simulink model "Haptic feedbck system"  (R2024b)
settings: Solver=ode4  StartTime=0.0  StopTime=inf  FixedStep=0.001  RelTol=1e-3  EnableMultiTasking=on
undefined symbols (not defined in the file): _, cablePTstudyZF, data, date, DiscIntNeverNeededParam, FETau, HIL, i2tTimeLim, iCmd2Volt, iCmdLim, iCmdSat, iCont, iMeasLim, iMeasServoConv, iPeak, iSign, kDposStudyPC, kDstudyZF, kPposStudyPC, kPstudyZF, kS, magnitude, maxTorque, motEncCnts2Rad, motEncSign, motKt, motNegFfTauStudyPC, motPosFfTauStudyPC, motPulleyRad, pulseGuiPeriod, pulseGuiPulseWidth, qc_get_step_size, signals, sprEncCnts2Rad, sprEncSign, tauDzStudyZF, tauJlim, tauMlim, tauNoMvtStudyZF, test_1_robot_torque_, time, tS, Visualization, xJdotLim, xJlimNeg, xJlimPos, xMdotLim, xMlimNeg, xMlimPos
libraries: quarc_library x26, simulink x13, simulink_extras x2
(part 1 of 3)
settings Model: SimulationMode=external  ExtModeTrigDuration=10000  Creator=Pranav  LastModifiedBy=Pranav
settings SolverCC: AlgebraicLoopSolver=TrustRegion  PositivePriorityOrder=on
settings DataIOCC: ReturnWorkspaceOutputs=off
settings DebuggingCC: UnconnectedInputMsg=warning  UnconnectedOutputMsg=warning  UnconnectedLineMsg=warning  ArithmeticOperatorsInVariantConditions=warning
settings ModelReferenceCC: EnableRefExpFcnMdlSchedulingChecks=on
settings SFSimCC: SimUseLocalCustomCode=off  CustomCodeUndefinedFunction=UseInterfaceOnly
settings RTWCC: Description=QUARC Win64 Target Using Toolchain  SystemTargetFile=quarc_win64.tlc  TemplateMakefile=quarc_default_tmf  RTWUseLocalCustomCode=off  Toolchain=QUARC win64 | nmake (64-bit Windows)  BuildConfiguration=Faster Runs  GPUComputeCapability=3.5
settings CodeAppCC: StateflowObjectComments=on
settings STFCustomTargetCC: TargetLangStandard=C99 (ISO)  ConcurrentExecutionCompliant=on  GRTInterface=on  UseToolchainInfoCompliant=on  SystemTargetFile=quarc_win64.tlc
settings GRTTargetCC: ParMdlRefBuildCompliant=off  CompOptLevelCompliant=off  CombineOutputUpdateFcns=off  MatFileLogging=off  CPPClassGenCompliant=off  GRTInterface=on  ExtMode=on  ExtModeMexFile=quarc_comm
settings ConfigComp: CovMetricSettings=dswe

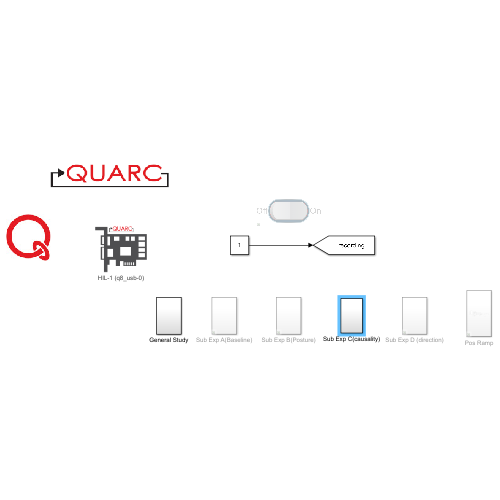
[thumbnail: Simulink's stored preview of the top-level diagram]
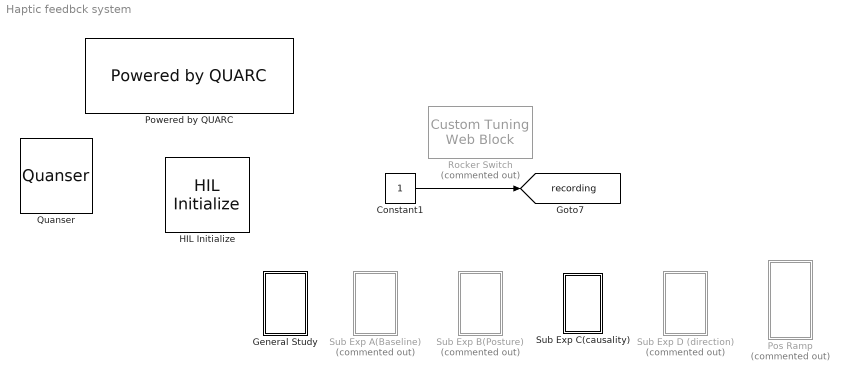
== system Haptic feedbck system ==
  Constant1 : Constant
  General Study : Subsystem
  HIL Initialize : quarc_library/Data Acquisition/Generic/Configuration/HIL Initialize  Priority=-99  object_name=HIL-1  board_type=q8_usb  board_number=0  board_options=update_rate=normal;decimation=1  exclusive=off  active=off  hardware_clocks=[0:2]  clock_modes=[]  initial_clock_frequencies=[]  set_clock_params_at_start=off  set_clock_params_at_switch_in=off  set_clock_frequencies_at_start=off  set_clock_frequencies_at_switch_in=off  analog_input_channels=[0:7]  analog_input_configurations=[]  analog_input_maximums=10  analog_input_minimums=-10  set_analog_input_params_at_start=on  set_analog_input_params_at_switch_in=off  analog_output_channels=[0:7]  analog_output_maximums=10  analog_output_minimums=-10  initial_analog_outputs=[0]  final_analog_outputs=[0]  watchdog_analog_outputs=0  set_analog_output_params_at_start=on  set_analog_output_params_at_switch_in=off  set_analog_outputs_at_start=on  set_analog_outputs_at_switch_in=off  set_analog_outputs_at_terminate=on  set_analog_outputs_at_switch_out=off  set_analog_outputs_on_watchdog=off  digital_input_channels=[]  digital_output_channels=0:7  digital_output_configuration=[]  initial_digital_outputs=[1]  final_digital_outputs=[1]  watchdog_digital_outputs=[0]  set_digital_output_params_at_start=off  set_digital_output_params_at_switch_in=off  set_digital_outputs_at_start=on  set_digital_outputs_at_switch_in=off  set_digital_outputs_at_terminate=on  set_digital_outputs_at_switch_out=off  set_digital_outputs_on_watchdog=off  encoder_channels=[0:7]  quadrature=[4]  encoder_filter_frequency=[]  initial_encoder_counts=[0]  set_encoder_params_at_start=on  set_encoder_params_at_switch_in=off  set_encoder_counts_at_start=off  set_encoder_counts_at_switch_in=off  pwm_channels=[0:7]  pwm_modes=0  pwm_frequency=99.532799999999995e6/4095  pwm_configuration=[0]  pwm_alignment=[0]  pwm_polarity=[1]  pwm_leading_deadband=[0]  pwm_trailing_deadband=[0]  initial_pwm_outputs=[0]  final_pwm_outputs=[0]  watchdog_pwm_outputs=[0]  set_pwm_params_at_start=on  set_pwm_params_at_switch_in=off  set_pwm_outputs_at_start=on  set_pwm_outputs_at_switch_in=off  set_pwm_outputs_at_terminate=on  set_pwm_outputs_at_switch_out=off  set_pwm_outputs_on_watchdog=off  other_output_channels=[]  initial_other_outputs=[]  final_other_outputs=[]  watchdog_other_outputs=[]  set_other_outputs_at_start=off  set_other_outputs_at_switch_in=off  set_other_outputs_at_terminate=off  set_other_outputs_at_switch_out=off  set_other_outputs_on_watchdog=off
  Pos Ramp : Subsystem  Commented=on
  Powered by QUARC : quarc_library/Logos/Powered by QUARC
  Quanser : quarc_library/Logos/Quanser
  Rocker Switch : CustomTuningWebBlock  Commented=on  LabelPosition=Hide  ShowInitialText=on  Configuration="{\"components\":[{\"name\":\"CustomSwitchStateComponent\",\"settings\":{\"position\":[0,0,1,1],\"states\":[{\"HitRegion\":{\"position\":[0,0,0.5,1]},\"Image\":{\"position\":[0.13,0,1,0.75],\"size\":[1,0.75],\"src\":\"data:image\\/svg+xml;base64,PHN2ZyB4bWxucz0iaHR0cDovL3d3dy53My5vcmcvMjAwMC9zdmciIHhtbG5zOnhsaW5rPSJodHRwOi8vd3d3LnczLm9yZy8xOTk5L3hsaW5rIiB2aWV3Qm94PSIwIDAgNzUgMjQuOCI+PGRlZnM+PHN0eWxlPi5jbHMtMXtmaWxsOnVybCgjcmFkaWFsLWdyYWRpZW50KTt9LmNscy0ye2ZpbGw6dXJsKCNyYWRpYWwtZ3JhZGllbnQtMik7fS5jbHMtM3tzdHJva2U6I2IyMDAwMDtzdHJva2Utd2lkdGg6MC4yNXB4O2ZpbGw6dXJsKCNsaW5lYXItZ3JhZGllbnQpO30uY2xzLTR7ZmlsbDp1cmwoI2xpbmVhci1ncmFkaWVudC0yKTt9LmNs ...(+3576 chars)\",\"srcOrientation\":\"Right\"},\"Label\":{\"color\":[0.5019607843137255,0.5019607843137255,0.5019607843137255],\"icon\":{\"size\":[0,0],\"src\":[],\"srcOrientation\":\"Right\"},\"iconPlacement\":\"left\",\"opacity\":1,\"position\":[0.5,0.08],\"show\":true,\"text\":{\"content\":\"Off\",\"font\":\"Helvetica\"}},\"Value\":0},{\"HitRegion\":{\"position\":[0,0.5,0.5,1]},\"Image\":{\"position\":[0.13,0,1,0.75],\"size\":[1,0.75],\"src\":\"data:image\\/svg+xml;base64,PHN2ZyB4bWxucz0iaHR0cDovL3d3dy53My5vcmcvMjAwMC9zdmciIHhtbG5zOnhsaW5rPSJodHRwOi8vd3d3LnczLm9yZy8xOTk5L3hsaW5rIiB2aWV3Qm94PSIwIDAgNzUgMjQuOCI+PGRlZnM+PHN0eWxlPi5jbHMtMXtmaWxsOnVybCgjcmFkaWFsLWdyYWRpZW50KTt9LmNscy0ye2ZpbGw6dXJsKCNyYWRpYWwtZ3JhZGllbnQtMik7fS5jbHMtM3tzdHJva2U6I2IyMDAwMDtzdHJva2Utd2lkdGg6MC4yNXB4O2ZpbGw6dXJsKCNsaW5lYXItZ3JhZGllbnQpO30uY2xzLTR7ZmlsbDp1cmwoI2xpbmVhci1ncmFkaWVudC0yKTt9LmNs ...(+3520 chars)\",\"srcOrientation\":\"Right\"},\"Label\":{\"color\":[0.5019607843137255,0.5019607843137255,0.5019607843137255],\"icon\":{\"size\":[0,0],\"src\":[],\"srcOrientation\":\"Right\"},\"iconPlacement\":\"left\",\"opacity\":1,\"position\":[0.5,0.92],\"show\":true,\"text\":{\"content\":\"On\",\"font\":\"Helvetica\"}},\"Value\":1}]}},{\"name\":\"BackgroundImageComponent\",\"settings\":{\"image\":{\"size\":[155,70],\"src\":\"default\",\"srcOrientation\":\"Right\"},\"position\":[0,0,1,1],\"scaleMode\":\"0\"}},{\"name\":\"ForegroundImageComponent\",\"settings\":{\"image\":{\"size\":[0,0],\"src\":\"default\",\"srcOrientation\":[]},\"isForeground\":1,\"position\":[0,0,1,1],\"scaleMode\":\"0\"}}],\"settings\":{\"BindingType\":\"param\",\"backgroundColor\":[0,0,255,\"1\"],\"backgroundOffset\":0.14,\"fixedAspectRatio\":\"on\",\"foregroundColor\":[234,234,234],\"showBackgroundColor\":false,\"variant\":\"rocker\",\"version\":\"R2024b\"},\"type\":\"Switch\"}"
  Sub Exp A(Baseline) : Subsystem  Commented=on
  Sub Exp B(Posture) : Subsystem  Commented=on
  Sub Exp C(causality) : Subsystem
  Sub Exp D (direction) : Subsystem  Commented=on
  tag scope: recording=global
  wires:
  Constant1/1 -> [recording]

== system Haptic feedbck system/General Study ==
  Calculations : Subsystem
  Enable : Subsystem
  Hardware Enable : Subsystem
  Measurements : Subsystem
  Simulation Stops : Subsystem

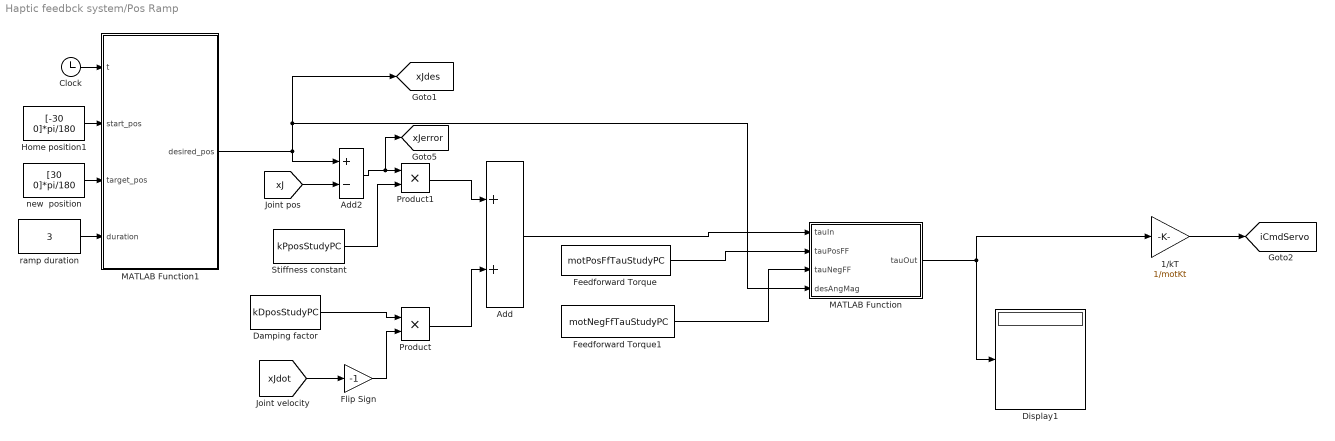
== system Haptic feedbck system/Pos Ramp ==
  1/kT : Gain  Gain=1/motKt
  Add : Sum
  Add2 : Sum  Inputs=+-
  Clock : Clock
  Damping factor : Constant  Value=kDposStudyPC
  Display1 : Display
  Feedforward Torque : Constant  Value=motPosFfTauStudyPC
  Feedforward Torque1 : Constant  Value=motNegFfTauStudyPC
  Flip Sign : Gain  Gain=-1
  Home position1 : Constant  Value=[-30 0]*pi/180
  MATLAB Function : MATLAB Function  TreatAsAtomicUnit=on
  MATLAB Function1 : MATLAB Function  TreatAsAtomicUnit=on
  Product : Product  RndMeth=Zero
  Product1 : Product  RndMeth=Zero
  Stiffness constant : Constant  Value=kPposStudyPC
  new  position : Constant  Value=[30 0]*pi/180
  ramp duration : Constant  Value=3
  tag scope: iCmdServo=global, xJdes=global, xJerror=global
  wires:
  Add2/1 -> [xJerror], Product1/1
  Damping factor/1 -> Product/1
  1/kT/1 -> [iCmdServo]
  Stiffness constant/1 -> Product1/2
  MATLAB Function/1(tauOut) -> Display1/1, 1/kT/1
  Flip Sign/1 -> Product/2
  [xJ] -> Add2/2
  [xJdot] -> Flip Sign/1
  Feedforward Torque1/1 -> MATLAB Function/3(tauNegFF)
  Feedforward Torque/1 -> MATLAB Function/2(tauPosFF)
  Add/1 -> MATLAB Function/1(tauIn)
  Product1/1 -> Add/1
  Product/1 -> Add/2
  MATLAB Function1/1(desired_pos) -> [xJdes], MATLAB Function/4(desAngMag), Add2/1
  new  position/1 -> MATLAB Function1/3(target_pos)
  Clock/1 -> MATLAB Function1/1(t)
  ramp duration/1 -> MATLAB Function1/4(duration)
  Home position1/1 -> MATLAB Function1/2(start_pos)

== system Haptic feedbck system/Sub Exp A(Baseline) ==
  "Active User Control " : Subsystem
  Active User GUI : Subsystem
  Active UserData Recording : Subsystem

== system Haptic feedbck system/Sub Exp B(Posture) ==
  "Active User Control " : Subsystem
  Active User GUI : Subsystem
  Active UserData Recording : Subsystem

== system Haptic feedbck system/Sub Exp C(causality) ==
  Passive User Control : Subsystem
  Passive User GUI : Subsystem
  Passive UserData Recording : Subsystem

== system Haptic feedbck system/Sub Exp D (direction) ==
  "Active User Control " : Subsystem
  Active User GUI : Subsystem
  Active UserData Recording : Subsystem

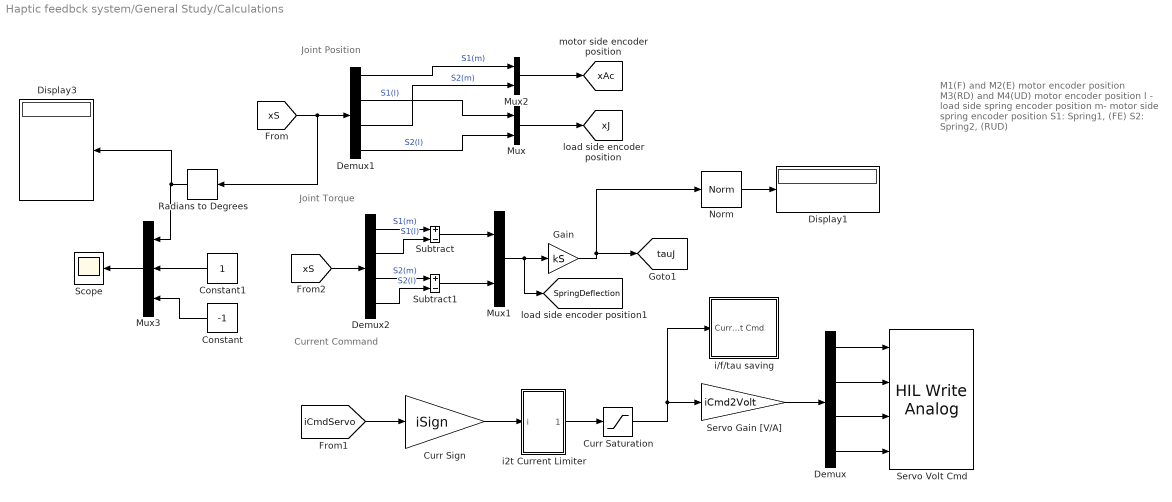
== system Haptic feedbck system/General Study/Calculations ==
  note: M1(F) and M2(E) motor encoder position
      | M3(RD) and M4(UD) motor encoder position
      | l - load side spring encoder position
      | m- motor side spring encoder position
      | S1: Spring1, (FE)
      | S2: Spring2, (RUD)
  note: Joint Position
  note: Joint Torque
  note: Current Command
  Constant : Constant  Value=-1
  Constant1 : Constant
  Curr Saturation : Saturate  UpperLimit=iCmdSat  LowerLimit=-iCmdSat
  Curr Sign : Gain  Gain=iSign
  Demux : Demux
  Demux1 : Demux
  Demux2 : Demux
  Display1 : Display
  Display3 : Display
  Gain : Gain  Gain=kS
  Mux : Mux  Inputs=2
  Mux1 : Mux  Inputs=2
  Mux2 : Mux  Inputs=2
  Mux3 : Mux  Inputs=3
  Norm : quarc_library/Math Operations/Vectors/Norm
      settings: SourceProductName=QUARC Targets
  Radians to Degrees : simulink_extras/Transformations/Radians to Degrees
  Scope : Scope
  Servo Gain [V/A] : Gain  Gain=iCmd2Volt
  Servo Volt Cmd : quarc_library/Data Acquisition/Generic/Immediate I//O/HIL Write Analog  object_name=HIL-1  channels=0:3  sample_time=-1  active=off  vector_input=off
  Subtract : Sum  Inputs=+-
  Subtract1 : Sum  Inputs=+-
  i/f/tau saving : Subsystem
  i2t Current Limiter : Subsystem
  tag scope: SpringDeflection=global, tauJ=global, xAc=global, xJ=global
  wires:
  [xS] -> Radians to Degrees/1, Demux1/1
  Demux1/2 -> Mux/1  "S1(l)"
  Demux1/1 -> Mux2/1  "S1(m)"
  Demux1/4 -> Mux/2  "S2(l)"
  [xS] -> Demux2/1
  Demux2/1 -> Subtract/1  "S1(m)"
  Demux2/2 -> Subtract/2  "S1(l)"
  Demux2/3 -> Subtract1/1  "S2(m)"
  Demux2/4 -> Subtract1/2  "S2(l)"
  Mux1/1 -> [SpringDeflection], Gain/1
  Gain/1 -> Norm/1, [tauJ]
  Demux/1 -> Servo Volt Cmd/1
  Servo Gain [V/A]/1 -> Demux/1
  Curr Saturation/1 -> Servo Gain [V/A]/1, i/f/tau saving/1(Current Cmd)
  Curr Sign/1 -> i2t Current Limiter/1(i)
  Demux/2 -> Servo Volt Cmd/2
  i2t Current Limiter/1(i_lim) -> Curr Saturation/1
  Demux/3 -> Servo Volt Cmd/3
  Demux/4 -> Servo Volt Cmd/4
  Mux/1 -> [xJ]
  Constant1/1 -> Mux3/2
  Mux3/1 -> Scope/1
  Norm/1 -> Display1/1
  Radians to Degrees/1 -> Display3/1, Mux3/1
  Demux1/3 -> Mux2/2  "S2(m)"
  Mux2/1 -> [xAc]
  Subtract/1 -> Mux1/1
  Subtract1/1 -> Mux1/2
  Constant/1 -> Mux3/3
  [iCmdServo] -> Curr Sign/1

== system Haptic feedbck system/General Study/Enable ==
  note: Enable (1 = On, 0 = Off)
  M1 Enable : Constant
  M2 Enable : Constant
  M3 Enable : Constant
  M4 Enable : Constant
  Master  Enable : Constant
  tag scope: M1Enable=global, M2Enable=global, M3Enable=global, M4Enable=global, masterEnable=global
  wires:
  M1 Enable/1 -> [M1Enable]
  Master  Enable/1 -> [masterEnable]
  M2 Enable/1 -> [M2Enable]
  M3 Enable/1 -> [M3Enable]
  M4 Enable/1 -> [M4Enable]

== system Haptic feedbck system/General Study/Hardware Enable ==
  note: Enable/Inhibit Hardware on Servo Amp
      | 0 = Off (GND)
      | 1 = On (+5v)
  note: Hardware Enable
  Gain{1..4} (4 alike) : Gain  Gain=5
  HIL Write Analog : quarc_library/Data Acquisition/Generic/Immediate I//O/HIL Write Analog  object_name=HIL-1  channels=4:7  sample_time=-1  active=off  vector_input=off
  Product{1..4} (4 alike) : Product  RndMeth=Zero
  Saturation{1..4} (4 alike) : Saturate  UpperLimit=5  LowerLimit=0
  wires:
  [M1Enable] -> Product1/1
  Product1/1 -> Gain1/1
  Product2/1 -> Gain2/1
  Saturation1/1 -> HIL Write Analog/1
  Saturation2/1 -> HIL Write Analog/2
  Gain1/1 -> Saturation1/1
  Gain2/1 -> Saturation2/1
  [M2Enable] -> Product2/1
  Product3/1 -> Gain3/1
  Saturation3/1 -> HIL Write Analog/3
  Gain3/1 -> Saturation3/1
  [M3Enable] -> Product3/1
  Product4/1 -> Gain4/1
  Saturation4/1 -> HIL Write Analog/4
  Gain4/1 -> Saturation4/1
  [M4Enable] -> Product4/1
  [masterEnable] -> Product4/2, Product3/2, Product2/2, Product1/2

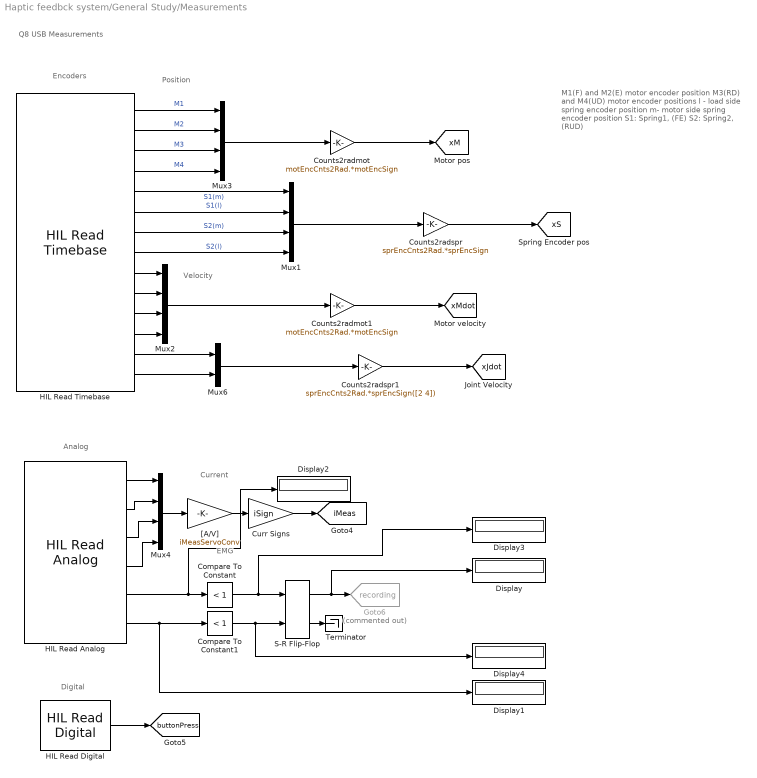
== system Haptic feedbck system/General Study/Measurements ==
  note: M1(F) and M2(E) motor encoder position
      | M3(RD) and M4(UD) motor encoder positions
      | l - load side spring encoder position
      | m- motor side spring encoder position
      | S1: Spring1, (FE)
      | S2: Spring2, (RUD)
  note: Current
  note: Q8 USB Measurements
  note: Encoders
  note: Digital
  note: EMG
  note: Analog
  note: Position
  note: Velocity
  Compare To Constant : simulink/Logic and Bit Operations/Compare To Constant  relop=<  const=1  OutDataTypeStr=boolean
  Compare To Constant1 : simulink/Logic and Bit Operations/Compare To Constant  relop=<  const=1  OutDataTypeStr=boolean
  Counts2radmot : Gain  Gain=motEncCnts2Rad.*motEncSign
  Counts2radmot1 : Gain  Gain=motEncCnts2Rad.*motEncSign
  Counts2radspr : Gain  Gain=sprEncCnts2Rad.*sprEncSign
  Counts2radspr1 : Gain  Gain=sprEncCnts2Rad.*sprEncSign([2 4])
  Curr Signs : Gain  Gain=iSign
  Display{,1..4} (5 alike) : Display
  Goto6 : Goto  Commented=on  GotoTag=recording  TagVisibility=global
  HIL Read Timebase : quarc_library/Data Acquisition/Generic/Timebases/HIL Read Timebase  object_name=HIL-1  clock=0  analog_channels=[]  encoder_channels=[0:7]  digital_channels=[]  other_channels=[14000:14003 14005 14007]  active=on  vector_output=off  data_type_mode=Inherit via back propagation  encoder_data_type=double  digital_data_type=boolean  overflow_mode=Error on overflow  samples_in_buffer=max(ceil(1/qc_get_step_size), 1)
  HIL Read Analog : quarc_library/Data Acquisition/Generic/Immediate I//O/HIL Read Analog  object_name=HIL-1  channels=[0:5]  sample_time=qc_get_step_size  active=on  vector_output=off
  HIL Read Digital : quarc_library/Data Acquisition/Generic/Immediate I//O/HIL Read Digital  object_name=HIL-1  channels=7  sample_time=qc_get_step_size  active=on  vector_output=off  data_type_mode=Inherit via back propagation  data_type=boolean
      settings: AttributesFormatString=(%<object_name>)  SourceProductName=QUARC Targets
  Mux{1..4} (4 alike) : Mux
  Mux6 : Mux  Inputs=2
  S-R Flip-Flop : simulink_extras/Flip Flops/S-R Flip-Flop  initial_condition=0
  Terminator : Terminator
  "[A/V]" : Gain  Gain=iMeasServoConv
  tag scope: buttonPress=global, iMeas=global, xJdot=global, xM=global, xMdot=global, xS=global
  wires:
  Mux3/1 -> Counts2radmot/1
  Counts2radspr/1 -> [xS]
  Counts2radmot/1 -> [xM]
  Mux4/1 -> "[A/V]"/1
  Curr Signs/1 -> [iMeas]
  "[A/V]"/1 -> Curr Signs/1
  HIL Read Analog/1 -> Mux4/1
  HIL Read Analog/2 -> Mux4/2
  HIL Read Analog/3 -> Mux4/3
  HIL Read Analog/4 -> Mux4/4
  Counts2radmot1/1 -> [xMdot]
  Mux2/1 -> Counts2radmot1/1
  HIL Read Digital/1 -> [buttonPress]
  HIL Read Timebase/1 -> Mux3/1  "M1"
  HIL Read Timebase/2 -> Mux3/2  "M2"
  HIL Read Timebase/3 -> Mux3/3  "M3"
  HIL Read Timebase/4 -> Mux3/4  "M4"
  HIL Read Timebase/5 -> Mux1/1  "S1(m)"
  HIL Read Timebase/6 -> Mux1/2  "S1(l)"
  HIL Read Timebase/7 -> Mux1/3  "S2(m)"
  HIL Read Timebase/8 -> Mux1/4  "S2(l)"
  Mux1/1 -> Counts2radspr/1
  HIL Read Timebase/9 -> Mux2/1
  HIL Read Timebase/10 -> Mux2/2
  HIL Read Timebase/11 -> Mux2/3
  HIL Read Timebase/12 -> Mux2/4
  HIL Read Timebase/13 -> Mux6/1
  HIL Read Timebase/14 -> Mux6/2
  Mux6/1 -> Counts2radspr1/1
  Counts2radspr1/1 -> [xJdot]
  Compare To Constant1/1 -> Display4/1, S-R Flip-Flop/2
  HIL Read Analog/5 -> Display2/1, Compare To Constant/1
  S-R Flip-Flop/1 -> Display/1, Goto6/1
  Compare To Constant/1 -> Display3/1, S-R Flip-Flop/1
  S-R Flip-Flop/2 -> Terminator/1
  HIL Read Analog/6 -> Display1/1, Compare To Constant1/1

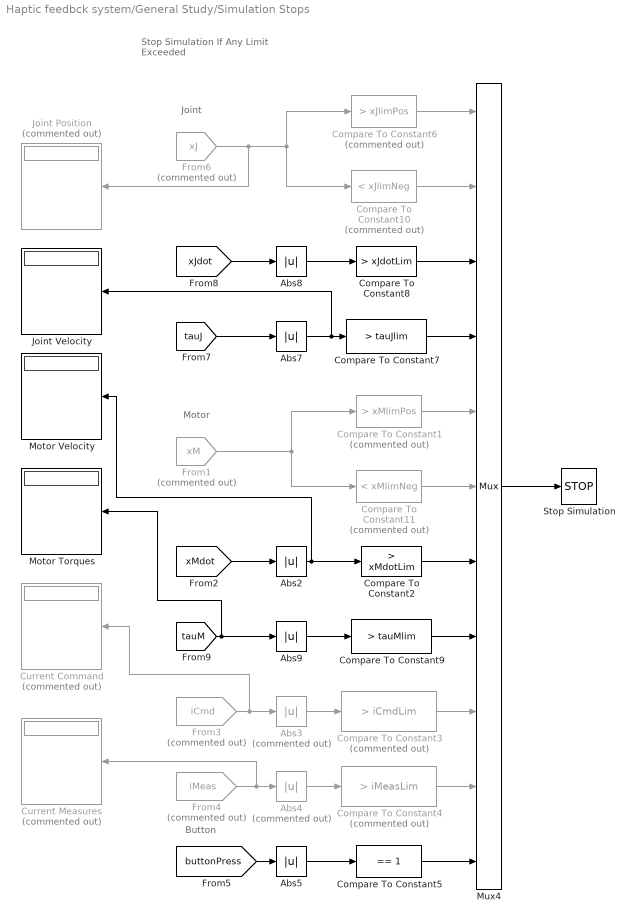
== system Haptic feedbck system/General Study/Simulation Stops ==
  note: Button
  note: Stop Simulation If Any
      | Limit Exceeded
  note: Motor
  note: Joint
  Abs{2,5,7..9} (5 alike) : Abs  SaturateOnIntegerOverflow=off
  Abs3 : Abs  Commented=on  SaturateOnIntegerOverflow=off
  Abs4 : Abs  Commented=on  SaturateOnIntegerOverflow=off
  Compare To Constant1 : simulink/Logic and Bit Operations/Compare To Constant  Commented=on  relop=>  const=xMlimPos  OutDataTypeStr=boolean
  Compare To Constant10 : simulink/Logic and Bit Operations/Compare To Constant  Commented=on  relop=<  const=xJlimNeg  OutDataTypeStr=boolean
  Compare To Constant11 : simulink/Logic and Bit Operations/Compare To Constant  Commented=on  relop=<  const=xMlimNeg  OutDataTypeStr=boolean
  Compare To Constant2 : simulink/Logic and Bit Operations/Compare To Constant  relop=>  const=xMdotLim  OutDataTypeStr=boolean
  Compare To Constant3 : simulink/Logic and Bit Operations/Compare To Constant  Commented=on  relop=>  const=iCmdLim  OutDataTypeStr=boolean
  Compare To Constant4 : simulink/Logic and Bit Operations/Compare To Constant  Commented=on  relop=>  const=iMeasLim  OutDataTypeStr=boolean
  Compare To Constant5 : simulink/Logic and Bit Operations/Compare To Constant  relop===  const=1  OutDataTypeStr=boolean
  Compare To Constant6 : simulink/Logic and Bit Operations/Compare To Constant  Commented=on  relop=>  const=xJlimPos  OutDataTypeStr=boolean
  Compare To Constant7 : simulink/Logic and Bit Operations/Compare To Constant  relop=>  const=tauJlim  OutDataTypeStr=boolean
  Compare To Constant8 : simulink/Logic and Bit Operations/Compare To Constant  relop=>  const=xJdotLim  OutDataTypeStr=boolean
  Compare To Constant9 : simulink/Logic and Bit Operations/Compare To Constant  relop=>  const=tauMlim  OutDataTypeStr=boolean
  Current Command : Display  Commented=on
  Current Measures : Display  Commented=on
  From1 : From  Commented=on  GotoTag=xM  TagVisibility=global
  From3 : From  Commented=on  GotoTag=iCmd  TagVisibility=global
  From4 : From  Commented=on  GotoTag=iMeas  TagVisibility=global
  From6 : From  Commented=on  GotoTag=xJ  TagVisibility=global
  Joint Position : Display  Commented=on
  Joint Velocity : Display
  Motor Torques : Display
  Motor Velocity : Display
  Mux4 : Mux  Inputs=11
  Stop Simulation : Stop
  wires:
  Abs5/1 -> Compare To Constant5/1
  [buttonPress] -> Abs5/1
  Abs3/1 -> Compare To Constant3/1
  From4/1 -> Current Measures/1, Abs4/1
  Abs4/1 -> Compare To Constant4/1
  From1/1 -> Compare To Constant11/1, Compare To Constant1/1
  [tauJ] -> Abs7/1
  Abs7/1 -> Joint Velocity/1, Compare To Constant7/1
  Abs8/1 -> Compare To Constant8/1
  [xJdot] -> Abs8/1
  [tauM] -> Abs9/1, Motor Torques/1
  Abs9/1 -> Compare To Constant9/1
  Abs2/1 -> Compare To Constant2/1, Motor Velocity/1
  [xMdot] -> Abs2/1
  From6/1 -> Joint Position/1, Compare To Constant6/1, Compare To Constant10/1
  Compare To Constant6/1 -> Mux4/1
  Compare To Constant10/1 -> Mux4/2
  Compare To Constant8/1 -> Mux4/3
  Compare To Constant7/1 -> Mux4/4
  Compare To Constant1/1 -> Mux4/5
  Compare To Constant11/1 -> Mux4/6
  Compare To Constant2/1 -> Mux4/7
  Compare To Constant9/1 -> Mux4/8
  Compare To Constant3/1 -> Mux4/9
  Compare To Constant4/1 -> Mux4/10
  Compare To Constant5/1 -> Mux4/11
  Mux4/1 -> Stop Simulation/1
  From3/1 -> Current Command/1, Abs3/1

== system Haptic feedbck system/Sub Exp A(Baseline)/Active User Control  ==
  1/kT : Gain  Gain=1/motKt
  Add : Sum
  Add2 : Sum  Inputs=+-
  Damping factor : Constant  Value=kDposStudyPC
  Display1 : Display
  Feedforward Torque : Constant  Value=motPosFfTauStudyPC
  Feedforward Torque1 : Constant  Value=motNegFfTauStudyPC
  Flip Sign : Gain  Gain=-1
  Home position1 : Constant  Value=[0 0]
  MATLAB Function : MATLAB Function  TreatAsAtomicUnit=on
  Product : Product  RndMeth=Zero
  Product1 : Product  RndMeth=Zero
  Stiffness constant : Constant  Value=kPposStudyPC
  tag scope: iCmdServo=global, xJdes=global, xJerror=global
  wires:
  Add2/1 -> [xJerror], Product1/1
  Damping factor/1 -> Product/1
  1/kT/1 -> [iCmdServo]
  Stiffness constant/1 -> Product1/2
  MATLAB Function/1(tauOut) -> Display1/1, 1/kT/1
  Flip Sign/1 -> Product/2
  [xJ] -> Add2/2
  [xJdot] -> Flip Sign/1
  Feedforward Torque1/1 -> MATLAB Function/3(tauNegFF)
  Feedforward Torque/1 -> MATLAB Function/2(tauPosFF)
  Add/1 -> MATLAB Function/1(tauIn)
  Product1/1 -> Add/1
  Product/1 -> Add/2
  Home position1/1 -> [xJdes], MATLAB Function/4(desAngMag), Add2/1

== system Haptic feedbck system/Sub Exp A(Baseline)/Active User GUI ==
  GUI Triggered Subsytem : Subsystem  TreatAsAtomicUnit=on
  Pulse Generator : DiscretePulseGenerator  PulseType=Time based  Period=pulseGuiPeriod  PulseWidth=pulseGuiPulseWidth
  target angles : Constant  Value=[0 180]*pi/180
  tag scope: FEtau2=global, RUtau2=global, TrialStart2=global, successfulTrial2=global, theta2=global
  wires:
  Pulse Generator/1 -> GUI Triggered Subsytem/Trigger
  target angles/1 -> GUI Triggered Subsytem/2(thetaSel)
  [tauJ] -> GUI Triggered Subsytem/1(tauJ)
  GUI Triggered Subsytem/1(Outport) -> [theta2]
  GUI Triggered Subsytem/2(Outport1) -> [FEtau2]
  GUI Triggered Subsytem/3(Outport2) -> [TrialStart2]
  GUI Triggered Subsytem/4(Outport3) -> [RUtau2]
  GUI Triggered Subsytem/5(Outport5) -> [successfulTrial2]

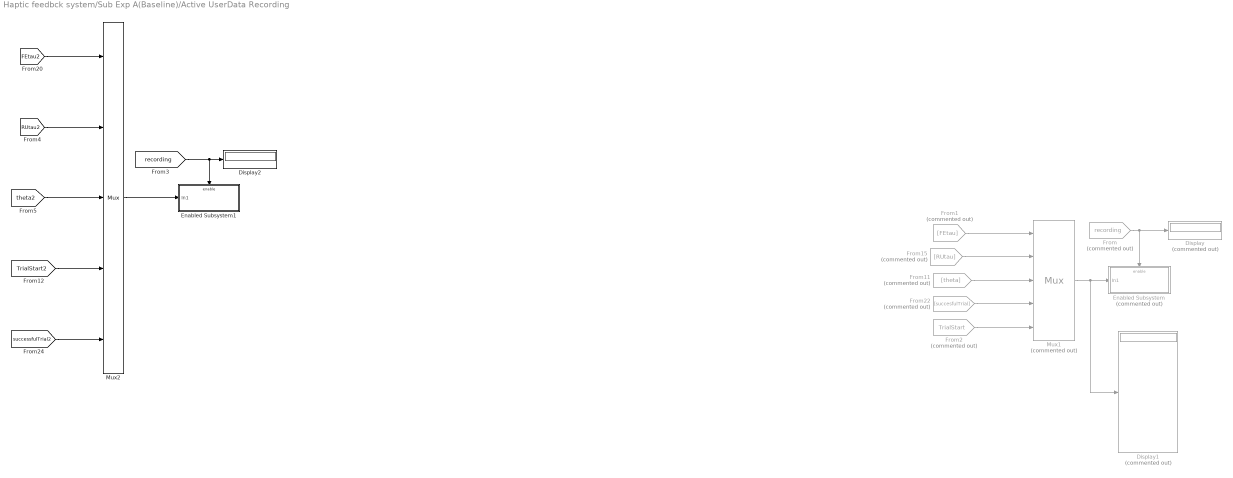
== system Haptic feedbck system/Sub Exp A(Baseline)/Active UserData Recording ==
  Display : Display  Commented=on
  Display1 : Display  Commented=on
  Display2 : Display
  Enabled Subsystem : Subsystem  Commented=on  TreatAsAtomicUnit=on
  Enabled Subsystem1 : Subsystem  TreatAsAtomicUnit=on
  From : From  Commented=on  GotoTag=recording  TagVisibility=global
  From1 : From  Commented=on  GotoTag=FEtau  TagVisibility=global
  From11 : From  Commented=on  GotoTag=theta  TagVisibility=global
  From15 : From  Commented=on  GotoTag=RUtau  TagVisibility=global
  From2 : From  Commented=on  GotoTag=TrialStart  TagVisibility=global
  From22 : From  Commented=on  GotoTag=succesfulTrial  TagVisibility=global
  Mux1 : Mux  Commented=on  Inputs=5
      settings: DisplayOption=signals
  Mux2 : Mux  Inputs=5
  wires:
  From/1 -> Display/1, Enabled Subsystem/Enable
  From1/1 -> Mux1/1
  From2/1 -> Mux1/5
  From15/1 -> Mux1/2
  From11/1 -> Mux1/3
  From22/1 -> Mux1/4
  Mux1/1 -> Display1/1, Enabled Subsystem/1(In1)
  [RUtau2] -> Mux2/2
  [recording] -> Display2/1, Enabled Subsystem1/Enable
  Mux2/1 -> Enabled Subsystem1/1(In1)
  [FEtau2] -> Mux2/1
  [theta2] -> Mux2/3
  [successfulTrial2] -> Mux2/5
  [TrialStart2] -> Mux2/4

== system Haptic feedbck system/Sub Exp B(Posture)/Active User Control  ==
  1/kT : Gain  Gain=1/motKt
  Add : Sum
  Add2 : Sum  Inputs=+-
  Damping factor : Constant  Value=kDposStudyPC
  Display1 : Display
  Feedforward Torque : Constant  Value=motPosFfTauStudyPC
  Feedforward Torque1 : Constant  Value=motNegFfTauStudyPC
  Flip Sign : Gain  Gain=-1
  Home position1 : Constant  Value=[-30 0]*pi/180
  MATLAB Function : MATLAB Function  TreatAsAtomicUnit=on
  Product : Product  RndMeth=Zero
  Product1 : Product  RndMeth=Zero
  Stiffness constant : Constant  Value=kPposStudyPC
  tag scope: iCmdServo=global, xJdes=global, xJerror=global
  wires:
  Add2/1 -> [xJerror], Product1/1
  Damping factor/1 -> Product/1
  1/kT/1 -> [iCmdServo]
  Stiffness constant/1 -> Product1/2
  MATLAB Function/1(tauOut) -> Display1/1, 1/kT/1
  Flip Sign/1 -> Product/2
  [xJ] -> Add2/2
  [xJdot] -> Flip Sign/1
  Feedforward Torque1/1 -> MATLAB Function/3(tauNegFF)
  Feedforward Torque/1 -> MATLAB Function/2(tauPosFF)
  Add/1 -> MATLAB Function/1(tauIn)
  Product1/1 -> Add/1
  Product/1 -> Add/2
  Home position1/1 -> [xJdes], MATLAB Function/4(desAngMag), Add2/1

== system Haptic feedbck system/Sub Exp B(Posture)/Active User GUI ==
  GUI Triggered Subsytem : Subsystem  TreatAsAtomicUnit=on
  Pulse Generator : DiscretePulseGenerator  PulseType=Time based  Period=pulseGuiPeriod  PulseWidth=pulseGuiPulseWidth
  target angles : Constant  Value=[0 180 0 180 0 180]*pi/180
  tag scope: FEtau2=global, RUtau2=global, TrialStart2=global, successfulTrial2=global, theta2=global
  wires:
  Pulse Generator/1 -> GUI Triggered Subsytem/Trigger
  target angles/1 -> GUI Triggered Subsytem/2(thetaSel)
  [tauJ] -> GUI Triggered Subsytem/1(tauJ)
  GUI Triggered Subsytem/1(Outport) -> [theta2]
  GUI Triggered Subsytem/2(Outport1) -> [FEtau2]
  GUI Triggered Subsytem/3(Outport2) -> [TrialStart2]
  GUI Triggered Subsytem/4(Outport3) -> [RUtau2]
  GUI Triggered Subsytem/5(Outport5) -> [successfulTrial2]

== system Haptic feedbck system/Sub Exp B(Posture)/Active UserData Recording ==
  Display2 : Display
  Enabled Subsystem1 : Subsystem  TreatAsAtomicUnit=on
  Mux2 : Mux  Inputs=5
  wires:
  [RUtau2] -> Mux2/2
  [recording] -> Display2/1, Enabled Subsystem1/Enable
  Mux2/1 -> Enabled Subsystem1/1(In1)
  [FEtau2] -> Mux2/1
  [theta2] -> Mux2/3
  [successfulTrial2] -> Mux2/5
  [TrialStart2] -> Mux2/4

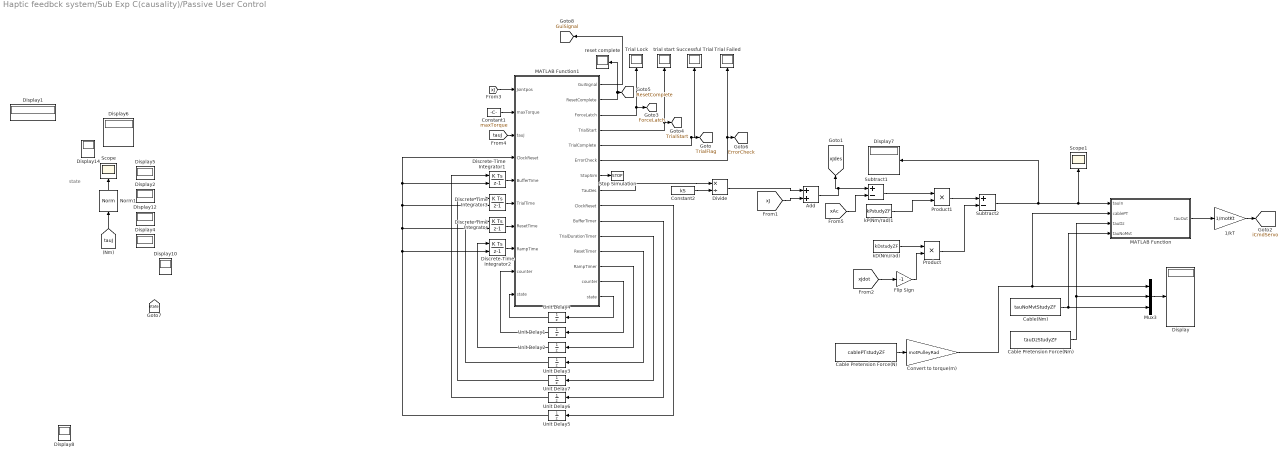
== system Haptic feedbck system/Sub Exp C(causality)/Passive User Control ==
  note: state
  1/kT : Gain  Gain=1/motKt
  Add : Sum
  Cable Pretension Force(N) : Constant  Value=cablePTstudyZF
  Cable Pretension Force(Nm) : Constant  Value=tauDzStudyZF
  Cable(Nm) : Constant  Value=tauNoMvtStudyZF
  Constant1 : Constant  Value=maxTorque
  Constant2 : Constant  Value=kS
  Convert to torque(m) : Gain  Gain=motPulleyRad
  Discrete-Time Integrator{,1..3} (4 alike) : DiscreteIntegrator  ExternalReset=rising  SampleTime=-1  ICPrevOutput=DiscIntNeverNeededParam  ICPrevScaledInput=DiscIntNeverNeededParam
  Display{,1..2,4..8,10,12,14} (11 alike) : Display
  Divide : Product  Inputs=*/
  Flip Sign : Gain  Gain=-1
  MATLAB Function : MATLAB Function  TreatAsAtomicUnit=on
  MATLAB Function1 : MATLAB Function  TreatAsAtomicUnit=on
  Mux3 : Mux  Inputs=3
  Norm1 : quarc_library/Math Operations/Vectors/Norm
      settings: SourceProductName=QUARC Targets
  Product : Product  RndMeth=Zero
  Product1 : Product  RndMeth=Zero
  Scope : Scope
  Scope1 : Scope
  Stop Simulation : Stop
  Subtract1 : Sum  Inputs=+-
  Subtract2 : Sum  Inputs=+-
  Successful Trial : Display
  Trial Failed : Display
  Trial Lock : Display
  Unit Delay{1..3,5..7} (6 alike) : UnitDelay  SampleTime=-1  HasFrameUpgradeWarning=on
  Unit Delay4 : UnitDelay  InitialCondition=1  SampleTime=-1  HasFrameUpgradeWarning=on
  kD(Nm/rad) : Constant  Value=kDstudyZF
  kP(Nm/rad)1 : Constant  Value=kPstudyZF
  reset complete : Display
  trial start : Display
  tag scope: ErrorCheck=global, ForceLatch=global, GuiSignal=global, ResetComplete=global, TrialFlag=global, TrialStart=global, iCmdServo=global, state=global, xJdes=global
  wires:
  [xJ] -> MATLAB Function1/1(Jointpos)
  [tauJ] -> Norm1/1
  Norm1/1 -> Scope/1
  Mux3/1 -> Display/1
  Cable(Nm)/1 -> Mux3/3, MATLAB Function/4(tauNoMvt)
  [xJdot] -> Flip Sign/1
  kD(Nm/rad)/1 -> Product/1
  Cable Pretension Force(N)/1 -> Convert to torque(m)/1
  MATLAB Function/1(tauOut) -> 1/kT/1
  Convert to torque(m)/1 -> Mux3/1, MATLAB Function/2(cablePT)
  Cable Pretension Force(Nm)/1 -> Mux3/2, MATLAB Function/3(tauDz)
  Flip Sign/1 -> Product/2
  Constant1/1 -> MATLAB Function1/2(maxTorque)
  Constant2/1 -> Divide/2
  Divide/1 -> Add/1
  [xJ] -> Add/2
  Add/1 -> Subtract1/1, [xJdes]
  Subtract1/1 -> Product1/1
  kP(Nm/rad)1/1 -> Product1/2
  Product1/1 -> Subtract2/1
  Product/1 -> Subtract2/2
  [xAc] -> Subtract1/2
  [tauJ] -> MATLAB Function1/3(tauJ)
  1/kT/1 -> [iCmdServo]
  Subtract2/1 -> Scope1/1, MATLAB Function/1(tauIn), Display7/1
  MATLAB Function1/7(StopSim) -> Stop Simulation/1
  Unit Delay4/1 -> MATLAB Function1/10("state ")
  MATLAB Function1/14(counter) -> Unit Delay1/1
  MATLAB Function1/13(RampTimer) -> Unit Delay2/1
  MATLAB Function1/12(ResetTimer) -> Unit Delay3/1
  MATLAB Function1/11(TrialDurationTimer) -> Unit Delay7/1
  MATLAB Function1/10(BufferTimer) -> Unit Delay6/1
  MATLAB Function1/9(ClockReset) -> Unit Delay5/1
  Unit Delay5/1 -> Discrete-Time Integrator/2, Discrete-Time Integrator1/2, MATLAB Function1/4("ClockReset "), Discrete-Time Integrator3/2, Discrete-Time Integrator2/2
  Discrete-Time Integrator2/1 -> MATLAB Function1/8(RampTime)
  Discrete-Time Integrator/1 -> MATLAB Function1/7(ResetTime)
  Discrete-Time Integrator3/1 -> MATLAB Function1/6(TrialTime)
  Discrete-Time Integrator1/1 -> MATLAB Function1/5(BufferTime)
  Unit Delay2/1 -> Discrete-Time Integrator2/1
  Unit Delay3/1 -> Discrete-Time Integrator/1
  Unit Delay7/1 -> Discrete-Time Integrator3/1
  Unit Delay6/1 -> Discrete-Time Integrator1/1
  MATLAB Function1/8(TauDes) -> Divide/1
  Unit Delay1/1 -> MATLAB Function1/9("counter ")
  MATLAB Function1/2(ResetComplete) -> [ResetComplete], reset complete/1
  MATLAB Function1/3(ForceLatch) -> Trial Lock/1, [ForceLatch]
  MATLAB Function1/4(TrialStart) -> trial start/1, [TrialStart]
  MATLAB Function1/5(TrialComplete) -> [TrialFlag], Successful Trial/1
  MATLAB Function1/6(ErrorCheck) -> [ErrorCheck], Trial Failed/1
  MATLAB Function1/15(state) -> Unit Delay4/1
  MATLAB Function1/1(GuiSignal) -> [GuiSignal]

== system Haptic feedbck system/Sub Exp C(causality)/Passive User GUI ==
  GUI Triggered Subsytem : Subsystem  TreatAsAtomicUnit=on
  Pulse Generator : DiscretePulseGenerator  PulseType=Time based  Period=pulseGuiPeriod  PulseWidth=pulseGuiPulseWidth
  tag scope: FEtau3=global, RUtau3=global, count=global, theta3=global
  wires:
  Pulse Generator/1 -> GUI Triggered Subsytem/Trigger
  [tauJ] -> GUI Triggered Subsytem/1(tauJ)
  GUI Triggered Subsytem/1(Outport) -> [theta3]
  GUI Triggered Subsytem/2(Outport1) -> [FEtau3]
  GUI Triggered Subsytem/3(Outport3) -> [RUtau3]
  [xJ] -> GUI Triggered Subsytem/6(Jointpos)
  [TrialFlag] -> GUI Triggered Subsytem/5(TrialFlag)
  GUI Triggered Subsytem/4(Outport4) -> [count]
  [ResetComplete] -> GUI Triggered Subsytem/4(Reset Complete)
  [ErrorCheck] -> GUI Triggered Subsytem/2(In3)
  [TrialStart] -> GUI Triggered Subsytem/3(In2)
  [GuiSignal] -> GUI Triggered Subsytem/7(In8)

== system Haptic feedbck system/Sub Exp C(causality)/Passive UserData Recording ==
  Display2 : Display
  Enabled Subsystem1 : Subsystem  TreatAsAtomicUnit=on
  Mux2 : Mux  Inputs=5
  wires:
  [RUtau3] -> Mux2/2
  [recording] -> Display2/1, Enabled Subsystem1/Enable
  Mux2/1 -> Enabled Subsystem1/1(In1)
  [FEtau3] -> Mux2/1
  [theta3] -> Mux2/3
  [TrialFlag] -> Mux2/5
  [TrialStart] -> Mux2/4

== system Haptic feedbck system/Sub Exp D (direction)/Active User Control  ==
  1/kT : Gain  Gain=1/motKt
  Add : Sum
  Add2 : Sum  Inputs=+-
  Damping factor : Constant  Value=kDposStudyPC
  Display1 : Display
  Feedforward Torque : Constant  Value=motPosFfTauStudyPC
  Feedforward Torque1 : Constant  Value=motNegFfTauStudyPC
  Flip Sign : Gain  Gain=-1
  Home position1 : Constant  Value=[0 0]
  MATLAB Function : MATLAB Function  TreatAsAtomicUnit=on
  Product : Product  RndMeth=Zero
  Product1 : Product  RndMeth=Zero
  Stiffness constant : Constant  Value=kPposStudyPC
  tag scope: iCmdServo=global, xJdes=global, xJerror=global
  wires:
  Add2/1 -> [xJerror], Product1/1
  Damping factor/1 -> Product/1
  1/kT/1 -> [iCmdServo]
  Stiffness constant/1 -> Product1/2
  MATLAB Function/1(tauOut) -> Display1/1, 1/kT/1
  Flip Sign/1 -> Product/2
  [xJ] -> Add2/2
  [xJdot] -> Flip Sign/1
  Feedforward Torque1/1 -> MATLAB Function/3(tauNegFF)
  Feedforward Torque/1 -> MATLAB Function/2(tauPosFF)
  Add/1 -> MATLAB Function/1(tauIn)
  Product1/1 -> Add/1
  Product/1 -> Add/2
  Home position1/1 -> [xJdes], MATLAB Function/4(desAngMag), Add2/1

== system Haptic feedbck system/Sub Exp D (direction)/Active User GUI ==
  GUI Triggered Subsytem : Subsystem  TreatAsAtomicUnit=on
  Pulse Generator : DiscretePulseGenerator  PulseType=Time based  Period=pulseGuiPeriod  PulseWidth=pulseGuiPulseWidth
  target angles : Constant  Value=(0:30:150)*pi/180
  target angles1 : Constant  Value=(180:30:330)*pi/180
  tag scope: FEtau1=global, RUtau1=global, TrialStart1=global, successfulTrial1=global, theta1=global
  wires:
  Pulse Generator/1 -> GUI Triggered Subsytem/Trigger
  [tauJ] -> GUI Triggered Subsytem/1(tauJ)
  GUI Triggered Subsytem/1(Outport) -> [theta1]
  GUI Triggered Subsytem/2(Outport1) -> [FEtau1]
  GUI Triggered Subsytem/3(Outport2) -> [TrialStart1]
  GUI Triggered Subsytem/4(Outport3) -> [RUtau1]
  GUI Triggered Subsytem/5(Outport5) -> [successfulTrial1]
  target angles/1 -> GUI Triggered Subsytem/2(thetaSel)

== system Haptic feedbck system/Sub Exp D (direction)/Active UserData Recording ==
  Display2 : Display
  Enabled Subsystem1 : Subsystem  TreatAsAtomicUnit=on
  Mux2 : Mux  Inputs=5
  wires:
  [RUtau1] -> Mux2/2
  [recording] -> Display2/1, Enabled Subsystem1/Enable
  Mux2/1 -> Enabled Subsystem1/1(In1)
  [FEtau1] -> Mux2/1
  [theta1] -> Mux2/3
  [successfulTrial1] -> Mux2/5
  [TrialStart1] -> Mux2/4

== system Haptic feedbck system/General Study/Calculations/i//f//tau saving ==
  Current Cmd : Inport
  Curr Sign : Gain  Gain=iSign
  kT : Gain  Gain=motKt
  tag scope: iCmd=global, tauM=global
  wires:
  Curr Sign/1 -> kT/1, [iCmd]
  kT/1 -> [tauM]
  Current Cmd/1 -> Curr Sign/1

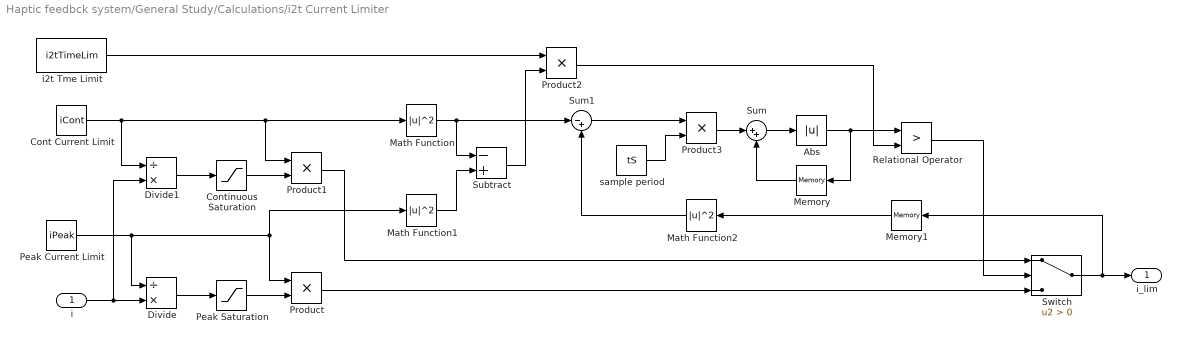
== system Haptic feedbck system/General Study/Calculations/i2t Current Limiter ==
  i : Inport
  Abs : Abs  SaturateOnIntegerOverflow=off
  Cont Current Limit : Constant  Value=iCont
  Continuous Saturation : Saturate  UpperLimit=1  LowerLimit=-1
  Divide : Product  Inputs=/*
  Divide1 : Product  Inputs=/*
  Math Function : Math  Operator=magnitude^2  SignedPower=on
  Math Function1 : Math  Operator=magnitude^2  SignedPower=on
  Math Function2 : Math  Operator=magnitude^2  SignedPower=on
  Memory : Memory
  Memory1 : Memory
  Peak Current Limit : Constant  Value=iPeak
  Peak Saturation : Saturate  UpperLimit=1  LowerLimit=-1
  Product{,1..3} (4 alike) : Product
  Relational Operator : RelationalOperator  Operator=>  OutDataTypeStr=boolean  InputSameDT=off
  Subtract : Sum  Inputs=-+
  Sum : Sum  Inputs=|++
  Sum1 : Sum  Inputs=|-+
  Switch : Switch  Criteria=u2 > Threshold  SaturateOnIntegerOverflow=off  InputSameDT=off
  i2t Tme Limit : Constant  Value=i2tTimeLim
  sample period : Constant  Value=tS
  i_lim : Outport
  wires:
  Memory1/1 -> Math Function2/1
  Abs/1 -> Memory/1, Relational Operator/1
  Relational Operator/1 -> Switch/2
  Product2/1 -> Relational Operator/2
  Product3/1 -> Sum/1
  sample period/1 -> Product3/2
  Sum1/1 -> Product3/1
  Math Function2/1 -> Sum1/2
  Sum/1 -> Abs/1
  Memory/1 -> Sum/2
  i2t Tme Limit/1 -> Product2/1
  Subtract/1 -> Product2/2
  Math Function1/1 -> Subtract/2
  Math Function/1 -> Subtract/1, Sum1/1
  Product1/1 -> Switch/1
  i/1 -> Divide1/2, Divide/2
  Cont Current Limit/1 -> Product1/1, Math Function/1, Divide1/1
  Continuous Saturation/1 -> Product1/2
  Divide1/1 -> Continuous Saturation/1
  Switch/1 -> i_lim/1, Memory1/1
  Product/1 -> Switch/3
  Peak Current Limit/1 -> Math Function1/1, Product/1, Divide/1
  Peak Saturation/1 -> Product/2
  Divide/1 -> Peak Saturation/1

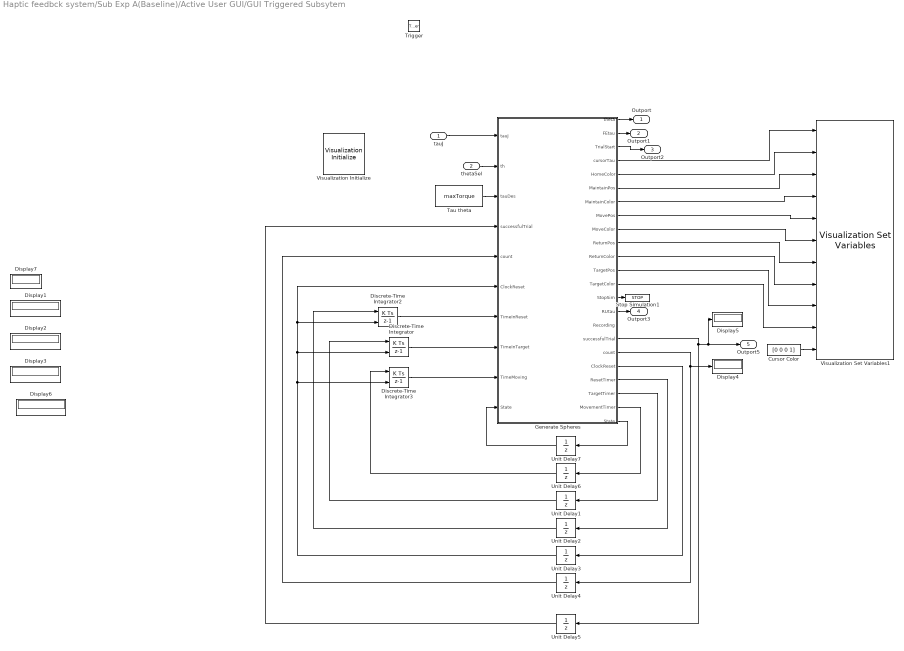
== system Haptic feedbck system/Sub Exp A(Baseline)/Active User GUI/GUI Triggered Subsytem ==
  tauJ : Inport
  thetaSel : Inport  Port=2
  Trigger : TriggerPort  VariantControl=(inherit)
  Cursor Color : Constant  Value=[0 0 0 1]  VectorParams1D=off
  Discrete-Time Integrator : DiscreteIntegrator  ExternalReset=rising  SampleTime=-1  OutDataTypeStr=double  ICPrevOutput=DiscIntNeverNeededParam  ICPrevScaledInput=DiscIntNeverNeededParam
  Discrete-Time Integrator2 : DiscreteIntegrator  ExternalReset=rising  SampleTime=-1  OutDataTypeStr=double  ICPrevOutput=DiscIntNeverNeededParam  ICPrevScaledInput=DiscIntNeverNeededParam
  Discrete-Time Integrator3 : DiscreteIntegrator  ExternalReset=rising  SampleTime=-1  OutDataTypeStr=double  ICPrevOutput=DiscIntNeverNeededParam  ICPrevScaledInput=DiscIntNeverNeededParam
  Display{1..7} (7 alike) : Display
  Generate Spheres : MATLAB Function  TreatAsAtomicUnit=on
  Stop Simulation1 : Stop
  Tau theta : Constant  Value=maxTorque  SampleTime=-1
  Unit Delay{1..6} (6 alike) : UnitDelay  SampleTime=-1  HasFrameUpgradeWarning=on
  Unit Delay7 : UnitDelay  InitialCondition=1  SampleTime=-1  StateName=State  HasFrameUpgradeWarning=on
  Visualization Initialize : quarc_library/User Interface/Visualization/Visualization Initialize  object_name=Visualization-1  scene_file=untitled.xml  uri=shmem://%m:1?private=visual  server_send_size=1000000  server_receive_size=1000  derive_from_server=on  client_send_size=1000  client_receive_size=1000000  variables=[ 20 24 34 40 44 50 54 60 64 70 74 ]  initial_values=single([ 0 0 0 1 1 1 1 1 1 1 1 -0.01 0 0 0 0 0 1 0 0 1 0 1 0 1 0 0 0 1 1 1 1 0 0 0 1 1 1 1 ])  open_on_start=on  close_on_stop=off
      settings: AttributesFormatString=%<object_name>  SourceProductName=QUARC Targets
  Visualization Set Variables1 : quarc_library/User Interface/Visualization/Visualization Set Variables  object_name=Visualization-1  offset=[ 11 7 32 35 0 3 25 28 18 21 14 ]  data_type=[ 0 0 0 0 0 0 0 0 0 0 0 ]  length=[ 3 4 3 4 3 4 3 4 3 4 4 ]  sample_time=visualization_get_frame_period  actor_name={'actor.cursor/Position';'actor.home/Diffuse Color';'actor.maintain/Position';'actor.maintain/Diffuse Color';'actor.move/Position';'actor.move/Diffuse Color';'actor.return/Position';'actor.return/Diffuse Color';'actor.target/Position';'actor.target/Diffuse Color';'actor.cursor/Diffuse Color'}
      settings: AttributesFormatString=(%<object_name>)  SourceProductName=QUARC Targets
  Outport : Outport
  Outport1 : Outport  Port=2
  Outport2 : Outport  Port=3
  Outport3 : Outport  Port=4
  Outport5 : Outport  Port=5
  wires:
  thetaSel/1 -> Generate Spheres/2(th)
  Tau theta/1 -> Generate Spheres/3(tauDes)
  tauJ/1 -> Generate Spheres/1(tauJ)
  Generate Spheres/19(ClockReset) -> Unit Delay3/1
  Generate Spheres/4(cursorTau) -> Visualization Set Variables1/1
  Generate Spheres/21(TargetTimer) -> Unit Delay1/1
  Unit Delay4/1 -> Generate Spheres/5("count ")
  Generate Spheres/17(successfulTrial) -> Display5/1, Outport5/1, Unit Delay5/1
  Unit Delay5/1 -> Generate Spheres/4("successfulTrial ")
  Unit Delay3/1 -> Generate Spheres/6("ClockReset "), Discrete-Time Integrator2/2, Discrete-Time Integrator/2, Discrete-Time Integrator3/2
  Generate Spheres/20(ResetTimer) -> Unit Delay2/1
  Discrete-Time Integrator3/1 -> Generate Spheres/9(TimeMoving)
  Generate Spheres/22(MovementTimer) -> Unit Delay6/1
  Unit Delay2/1 -> Discrete-Time Integrator2/1
  Discrete-Time Integrator2/1 -> Generate Spheres/7(TimeInReset)
  Unit Delay1/1 -> Discrete-Time Integrator/1
  Unit Delay6/1 -> Discrete-Time Integrator3/1
  Discrete-Time Integrator/1 -> Generate Spheres/8(TimeInTarget)
  Generate Spheres/23(State) -> Unit Delay7/1
  Generate Spheres/5(HomeColor) -> Visualization Set Variables1/2
  Generate Spheres/6(MaintainPos) -> Visualization Set Variables1/3
  Generate Spheres/7(MaintainColor) -> Visualization Set Variables1/4
  Generate Spheres/8(MovePos) -> Visualization Set Variables1/5
  Generate Spheres/9(MoveColor) -> Visualization Set Variables1/6
  Generate Spheres/10(ReturnPos) -> Visualization Set Variables1/7
  Generate Spheres/11(ReturnColor) -> Visualization Set Variables1/8
  Generate Spheres/12(TargetPos) -> Visualization Set Variables1/9
  Generate Spheres/13(TargetColor) -> Visualization Set Variables1/10
  Cursor Color/1 -> Visualization Set Variables1/11
  Generate Spheres/1(theta) -> Outport/1
  Generate Spheres/2(FEtau) -> Outport1/1
  Generate Spheres/3(TrialStart) -> Outport2/1
  Generate Spheres/15(RUtau) -> Outport3/1
  Generate Spheres/14(StopSim) -> Stop Simulation1/1
  Generate Spheres/18(count) -> Display4/1, Unit Delay4/1
  Unit Delay7/1 -> Generate Spheres/10("State ")

== system Haptic feedbck system/Sub Exp A(Baseline)/Active UserData Recording/Enabled Subsystem ==
  In1 : Inport
  Enable : EnablePort
  To Host File : quarc_library/Sinks/To Host/To Host File  source=Specify via dialog (do not evaluate)  file_name=test_1_robot_torque_%{date}_%{time}  variable_name=data%signals,data%FETau  decimation=1  sample_time=-1  file_format=CSV-file  options=Include header and footer  append=off  final_file_name=test_1_robot_torque_26-Sep-2025_11-47-39.csv  bitrate=2000000
  wires:
  In1/1 -> To Host File/1

== system Haptic feedbck system/Sub Exp A(Baseline)/Active UserData Recording/Enabled Subsystem1 ==
  In1 : Inport
  Enable : EnablePort
  To Host File : quarc_library/Sinks/To Host/To Host File  source=Specify via dialog (do not evaluate)  file_name=Main_study_p3_C1_R1  variable_name=data  decimation=1  sample_time=-1  file_format=CSV-file  options=Include header only  append=off  final_file_name=Main_study_p3_C1_R1.csv  bitrate=2000000
  wires:
  In1/1 -> To Host File/1
